simulink model "controlFuzzy"  (R2018b)
settings: Solver=VariableStepAuto  StartTime=0.0  StopTime=10.0  RelTol=1e-3
libraries: fuzblock x1
settings Model: Creator=ramon  LastModifiedBy=ramon

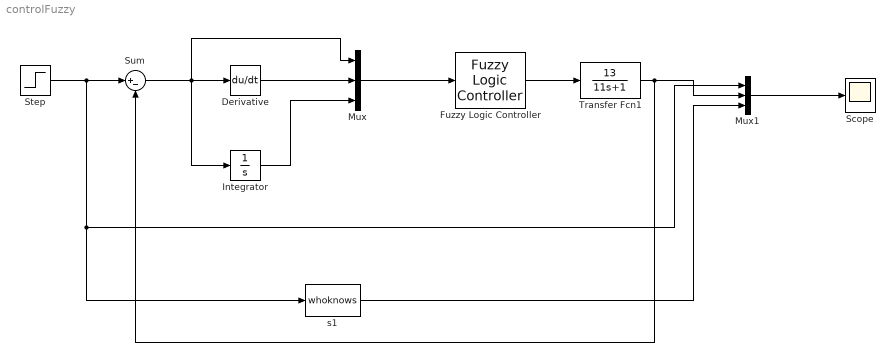
== system controlFuzzy ==
  Derivative : Derivative
  Fuzzy Logic Controller : fuzblock/Fuzzy Logic  Controller  FIS='tipper.fis'  OutputSampleNumber=101  DataType=double  FuzzifiedInputs=off  RuleFiringStrengths=off  RuleOutputs=off  AggregatedOutputs=off  SimulateUsing=Interpreted execution  OutOfRangeInputValueMessage=warning  NoRuleFiredMessage=warning  EmptyOutputFuzzySetMessage=warning
  Integrator : Integrator
  Mux : Mux  Inputs=3
  Mux1 : Mux  Inputs=3
  Scope : Scope
  Step : Step  SampleTime=0
  Sum : Sum  Inputs=|+-
  Transfer Fcn1 : TransferFcn  Numerator=13  Denominator=[11 1]
  s1 : M-S-Function  FunctionName=whoknows  Parameters=L, P1, P2, T, R  mask{L=7, P1=0, P2=9, T=1, R=0}
      mask prompts: L "Laboratorio"; P1 "Primer digito del Puesto"; P2 "Segundo digito del Puesto"; T "Tipo de Planta"; R "Ruido"
      mask Display: disp('Sistema')
  wires:
  Step/1 -> Mux1/1, s1/1, Sum/1
  Sum/1 -> Mux/1, Integrator/1, Derivative/1
  Integrator/1 -> Mux/3
  Derivative/1 -> Mux/2
  s1/1 -> Mux1/3
  Mux/1 -> Fuzzy Logic Controller/1
  Transfer Fcn1/1 -> Sum/2, Mux1/2
  Fuzzy Logic Controller/1 -> Transfer Fcn1/1
  Mux1/1 -> Scope/1
